simulink model "GradingSystem"  (R2021a)
settings: Solver=FixedStepDiscrete  StartTime=0.0  StopTime=10.0  RelTol=1e-3  EnableMultiTasking=on
settings Model: Creator=top one  LastModifiedBy=top one
settings DataIOCC: ReturnWorkspaceOutputs=off
settings OptimizationCC: DefaultParameterBehavior=Inlined  InlineInvariantSignals=on  EnableMemcpy=off  LifeSpan=1  EfficientTunableParamExpr=on
settings DebuggingCC: UnderspecifiedInitializationDetection=Classic  MergeDetectMultiDrivingBlocksExec=none  SFMachineParentedDataDiag=warning  ArithmeticOperatorsInVariantConditions=warning
settings ModelReferenceCC: PropagateSignalLabelsOutOfModel=off
settings SFSimCC: MATLABDynamicMemAlloc=off  CustomCodeUndefinedFunction=UseInterfaceOnly
settings RTWCC: SystemTargetFile=ert.tlc  GenCodeOnly=on  TemplateMakefile=ert_default_tmf  GenerateReport=on  IncludeHyperlinkInReport=on  LaunchReport=on  GenerateTraceInfo=on  GenerateTraceReport=on  GenerateTraceReportSl=on  GenerateTraceReportSf=on  GenerateTraceReportEml=on
settings CodeAppCC: ForceParamTrailComments=on  IgnoreCustomStorageClasses=off  OperatorAnnotations=on  SimulinkDataObjDesc=on  SFDataObjDesc=on  MATLABFcnDesc=on  InsertBlockDesc=on  StateflowObjectComments=on  MATLABSourceComments=on
settings ERTTargetCC: MultiwordLength=2048  GenerateSampleERTMain=on  InlinedParameterPlacement=NonHierarchical  ERTCustomFileTemplate=example_file_process.tlc

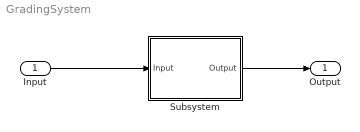
== system GradingSystem ==
  Input : Inport
  Subsystem : Subsystem
  Output : Outport
  wires:
  Input/1 -> Subsystem/1(Input)
  Subsystem/1(Output) -> Output/1

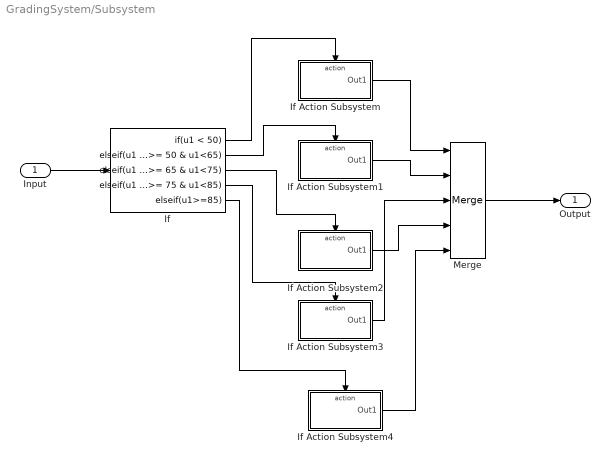
== system GradingSystem/Subsystem ==
  Input : Inport
  If : If  IfExpression=u1 < 50  ElseIfExpressions=u1 >= 50 & u1<65,u1 >= 65 & u1<75,u1 >= 75 & u1<85,u1>=85  ShowElse=off
  If Action Subsystem : Subsystem  TreatAsAtomicUnit=on
  If Action Subsystem1 : Subsystem  TreatAsAtomicUnit=on
  If Action Subsystem2 : Subsystem  TreatAsAtomicUnit=on
  If Action Subsystem3 : Subsystem  TreatAsAtomicUnit=on
  If Action Subsystem4 : Subsystem  TreatAsAtomicUnit=on
  Merge : Merge  Inputs=5
  Output : Outport
  wires:
  If Action Subsystem4/1(Out1) -> Merge/5
  If/3 -> If Action Subsystem2/Action
  If Action Subsystem/1(Out1) -> Merge/1
  If/5 -> If Action Subsystem4/Action
  If/1 -> If Action Subsystem/Action
  If/2 -> If Action Subsystem1/Action
  If Action Subsystem2/1(Out1) -> Merge/4
  If/4 -> If Action Subsystem3/Action
  Merge/1 -> Output/1
  If Action Subsystem3/1(Out1) -> Merge/3
  If Action Subsystem1/1(Out1) -> Merge/2
  Input/1 -> If/1

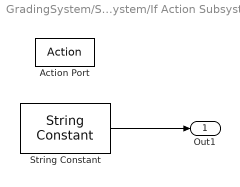
== system GradingSystem/Subsystem/If Action Subsystem ==
  Action Port : ActionPort  ActionPortLabel=if(u1 < 50)
  String Constant : StringConstant  String="\"Failed!\""
  Out1 : Outport
  wires:
  String Constant/1 -> Out1/1

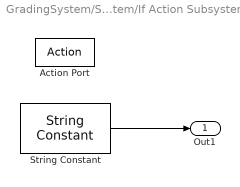
== system GradingSystem/Subsystem/If Action Subsystem1 ==
  Action Port : ActionPort  ActionPortLabel=elseif(u1 >= 50 & u1<65)
  String Constant : StringConstant  String="\"D\""
  Out1 : Outport
  wires:
  String Constant/1 -> Out1/1

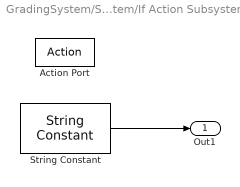
== system GradingSystem/Subsystem/If Action Subsystem2 ==
  Action Port : ActionPort  ActionPortLabel=elseif(u1 >= 65 & u1<75)
  String Constant : StringConstant  String="\"C\""
  Out1 : Outport
  wires:
  String Constant/1 -> Out1/1

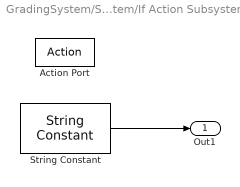
== system GradingSystem/Subsystem/If Action Subsystem3 ==
  Action Port : ActionPort  ActionPortLabel=elseif(u1 >= 75 & u1<85)
  String Constant : StringConstant  String="\"B\""
  Out1 : Outport
  wires:
  String Constant/1 -> Out1/1

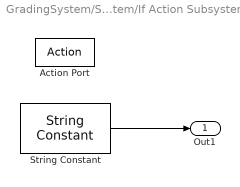
== system GradingSystem/Subsystem/If Action Subsystem4 ==
  Action Port : ActionPort  ActionPortLabel=elseif(u1>=85)
  String Constant : StringConstant  String="\"A\""
  Out1 : Outport
  wires:
  String Constant/1 -> Out1/1
